simulink model "PI2"  (R2020b)
settings: Solver=VariableStepAuto  StartTime=0.0  StopTime=10.0  RelTol=1e-3
model workspace (MAT data in the model file):
  Ki = Simulink.Parameter
  Ki.Value = 40
  Ki.DataType = 'auto'
  Ki.Dimensions = [1 1]
  Kp = Simulink.Parameter
  Kp.Value = 5000
  Kp.DataType = 'auto'
  Kp.Dimensions = [1 1]
settings Model: DataDictionary=Data_Dictionary.sldd  Creator=hp  LastModifiedBy=hp
settings DataIOCC: SaveOutput=off  SaveTime=off

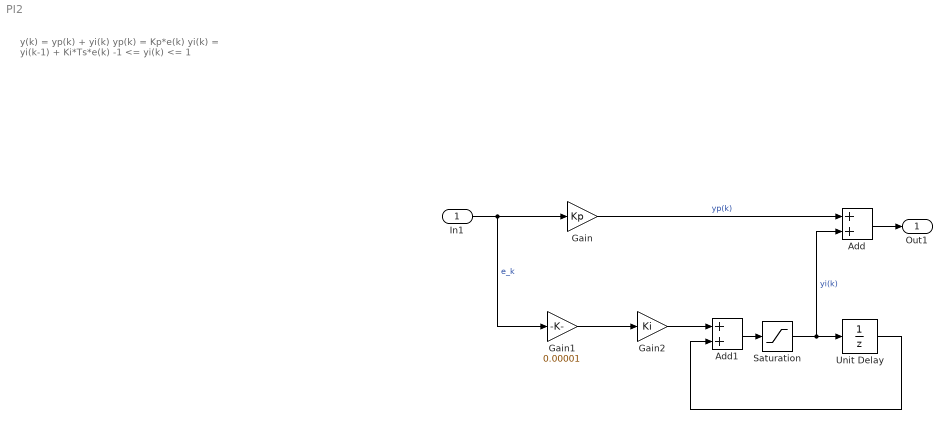
== system PI2 ==
  note: y(k) = yp(k) + yi(k)
      | yp(k) = Kp*e(k)
      | yi(k) = yi(k-1) + Ki*Ts*e(k)
      | -1 <= yi(k) <= 1
  In1 : Inport  OutDataTypeStr=double  PortDimensions=1  SampleTime=0
  Add : Sum
  Add1 : Sum
  Gain : Gain  Gain=Kp
  Gain1 : Gain  Gain=0.00001
  Gain2 : Gain  Gain=Ki
  Saturation : Saturate  UpperLimit=1  LowerLimit=-1
  Unit Delay : UnitDelay  SampleTime=-1  HasFrameUpgradeWarning=on
  Out1 : Outport  OutDataTypeStr=double  PortDimensions=1  SampleTime=0
  wires:
  Add/1 -> Out1/1
  Gain/1 -> Add/1  "yp(k)"
  Saturation/1 -> Unit Delay/1, Add/2  "yi(k)"
  Add1/1 -> Saturation/1
  Gain2/1 -> Add1/1
  In1/1 -> Gain/1, Gain1/1  "e_k"
  Gain1/1 -> Gain2/1
  Unit Delay/1 -> Add1/2
